simulink model "waterTankMdl"  (R2015a)
settings: Solver=ode45  StartTime=0.0  StopTime=final_time  RelTol=1e-6  AbsTol=1e-6
values from neighbouring files (symbols this model uses):
  A = 1    [Interacting_with_Simulink.m]    (also in population_model.m = [0     0.10 0.60 0.40 0.10 0.02 0.00 0.00 0.00)
  a = 1/2    (= 0.5)    [Euler_method.m]    (also in Interacting_with_Simulink.m = 0.02)
  g = 9.8    [Interacting_with_Simulink.m]
  h0 = 1    [Interacting_with_Simulink.m]
settings Model: Creator=PTMB  LastModifiedBy=PTMB

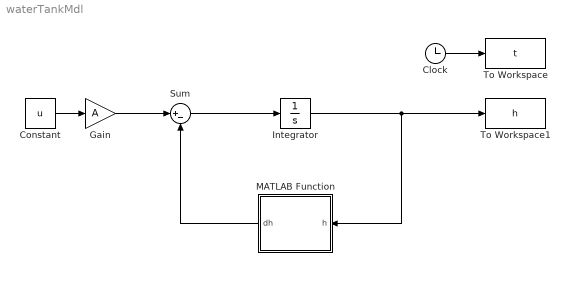
== system waterTankMdl ==
  Clock : Clock
  Constant : Constant  Value=u
  Gain : Gain  Gain=A
  Integrator : Integrator  InitialCondition=h0
  MATLAB Function : MATLAB Function  TreatAsAtomicUnit=on
  Sum : Sum  Inputs=|+-
  To Workspace : ToWorkspace  VariableName=t  SampleTime=-1
  To Workspace1 : ToWorkspace  VariableName=h  SampleTime=-1
  wires:
  Sum/1 -> Integrator/1
  MATLAB Function/1(dh) -> Sum/2
  Integrator/1 -> To Workspace1/1, MATLAB Function/1(h)
  Clock/1 -> To Workspace/1
  Constant/1 -> Gain/1
  Gain/1 -> Sum/1

== matlab function waterTankMdl/MATLAB Function ==
  data: h input; dh output; a parameter; A parameter; g parameter
function dh = fcn(h, a, A, g)
%#codegen

if (h > 0)
    dh = a * sqrt(2*g) / A * sqrt(h);
else
    dh = 0;
end
